simulink model "Simulink_tervezes"  (R2020b)
settings: Solver=VariableStepAuto  StartTime=0.0  StopTime=60  RelTol=1e-3
undefined symbols (not defined in the file): R, S, T, Ts
libraries: cstblocks x3
settings Model: Creator=kisel  LastModifiedBy=kisel

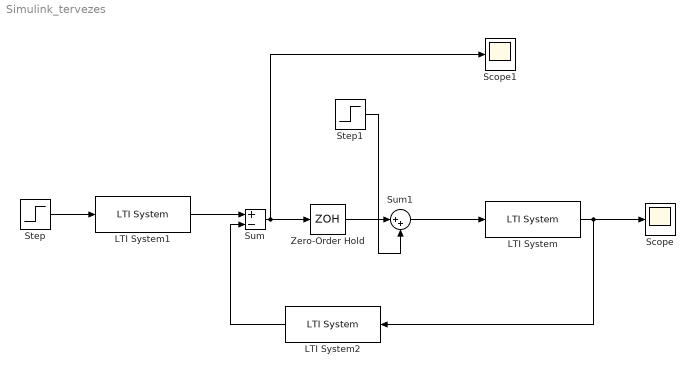
== system Simulink_tervezes ==
  LTI System : cstblocks/LTI System  sys=Wp  IC=[]
  LTI System1 : cstblocks/LTI System  sys=tf(T,R,Ts)  IC=[]
  LTI System2 : cstblocks/LTI System  sys=tf(S,R,Ts)  IC=[]
  Scope : Scope
  Scope1 : Scope
  Step : Step  Time=0  SampleTime=0
  Step1 : Step  Time=30  SampleTime=0
  Sum : Sum  Inputs=+-
  Sum1 : Sum  Inputs=|++
  Zero-Order Hold : ZeroOrderHold  SampleTime=Ts
  wires:
  LTI System1/1 -> Sum/1
  Step/1 -> LTI System1/1
  LTI System2/1 -> Sum/2
  LTI System/1 -> LTI System2/1, Scope/1
  Zero-Order Hold/1 -> Sum1/1
  Step1/1 -> Sum1/2
  Sum1/1 -> LTI System/1
  Sum/1 -> Scope1/1, Zero-Order Hold/1
